simulink library "LibEEPROM_eeprom_example_ORIGINAL"  (Simulink 10.0)
settings: Solver=VariableStepAuto  StartTime=0.0  StopTime=10.0  RelTol=1e-3
undefined symbols (not defined in the file): CRC32_calc_and_EEPROM_Write_ALL, crc32_calc_intern, CRC32_EEPROM_Read, EEPROM_Mirror, EEPROM_Read, IO_Blk_Lib_TTC500, IO_EEPROM_GetStatus, IO_EEPROM_Init, IO_EEPROM_Write, Read_Mirror, Write_Mirror, Write_Mirror_prepare_EEPROM
libraries: simulink x56
(part 7 of 8)

== system LibEEPROM_eeprom_example_ORIGINAL/EEPROM_WriteRetain/EEPROM_retain_var_1 ==
  note: NO IO_EEPROM_Write
      | perfomted here. This is
      | done in CRC32_calc_and_EEPROM_Write_ALL
  trigger : Inport
  data : Inport  Port=2  OutDataTypeStr=EEPROM_type
  Compare To Zero : simulink/Logic and Bit Operations/Compare To Zero  relop===  OutDataTypeStr=boolean  ZeroCross=off
  Compare To Zero1 : simulink/Logic and Bit Operations/Compare To Zero  relop=~=  OutDataTypeStr=boolean  ZeroCross=off
  Write_Mirror : Subsystem  LoadFcn=|  mask(Write_Mirror_Code){SampleTime=-1, ttlib=IO_Blk_Lib_TTC500, ttDescription=Write_Mirror, tt_iolib_version=0.19, offset=offset, length=length}
      | try
      | %
      | %Upgrade Information - standard BEGIN
      | new_color = 'blue';
      | new_ver = '0.19';
      | act_ver = get_param(gcb,'tt_iolib_version');
      | if not(strcmp(act_ver,new_ver))
      |     disp(['Upgrade block: ',gcb,char(10),'       Version: ',act_ver,' -> ',new_ver]);
      |     %switch - case for specific upgrade information e.g. additional parameter required 
      |     %Change appearance and version information
      |     set_param(gcb,'ForegroundColor',new_color);
      |     set_param(gcb,'tt_iolib_version',new_ver);
      | end
      | %Upgrade Information - standard END
      | catch
      | %Standard catch section BEGIN 
      | disp(' ');
      | disp('------------------------------------------------------------');
      | disp('An error occurred in a callback of the TTC580-BlockLib.');
      | disp('Please copy the following lines and report this to support@tttech.com ');
      | disp('<< begin of error message dump >>');
      | disp(['Version of TTC580-BlockLib: ', get_param(gcb,'tt_iolib_version')]);
      | disp(get_param(gcb,'ttDescription'));
      | disp(gcb);
      | x=lasterror;disp(x.message);
      | disp(get_param(gcb,'MaskValues'));
      | disp(version);
      | disp(computer);
      | disp('<< end of error message dump >>');
      | disp('------------------------------------------------------------');
      | disp(' ');
      | %Standard catch section END
      | end
      mask help:
      | Write data to the mirror of the EEPROM. ErrorCode is set to IO_E_BUSY for one cycle of writing into EEPROM_mirror[].
      | In case the given data section exceeds given EEPROM boundaries, IO_E_EEPROM_RANGE ErrorCode is returned.
      mask init:
      | %
      settings: CopyFcn=%deleted
      mask Help: web(which('~.h'))
      mask Callback offset: %
      mask Callback length: %
  b_ready : Outport  VectorParamsAs1DForOutWhenUnconnected=off
  wires:
  Compare To Zero1/1 -> Write_Mirror/1(b_trigger)
  Write_Mirror/1(ErrorCode_EEPROM_mirror) -> Compare To Zero/1
  data/1 -> Write_Mirror/2(data)
  trigger/1 -> Compare To Zero1/1
  Compare To Zero/1 -> b_ready/1

== system LibEEPROM_eeprom_example_ORIGINAL/EEPROM_WriteRetain/EEPROM_retain_var_2 ==
  note: NO IO_EEPROM_Write
      | perfomted here. This is
      | done in CRC32_calc_and_EEPROM_Write_ALL
  trigger : Inport
  data : Inport  Port=2  OutDataTypeStr=EEPROM_type
  Compare To Zero : simulink/Logic and Bit Operations/Compare To Zero  relop===  OutDataTypeStr=boolean  ZeroCross=off
  Compare To Zero1 : simulink/Logic and Bit Operations/Compare To Zero  relop=~=  OutDataTypeStr=boolean  ZeroCross=off
  Write_Mirror : Subsystem  LoadFcn=|  mask(Write_Mirror_Code){SampleTime=-1, ttlib=IO_Blk_Lib_TTC500, ttDescription=Write_Mirror, tt_iolib_version=0.19, offset=offset, length=length}
      | try
      | %
      | %Upgrade Information - standard BEGIN
      | new_color = 'blue';
      | new_ver = '0.19';
      | act_ver = get_param(gcb,'tt_iolib_version');
      | if not(strcmp(act_ver,new_ver))
      |     disp(['Upgrade block: ',gcb,char(10),'       Version: ',act_ver,' -> ',new_ver]);
      |     %switch - case for specific upgrade information e.g. additional parameter required 
      |     %Change appearance and version information
      |     set_param(gcb,'ForegroundColor',new_color);
      |     set_param(gcb,'tt_iolib_version',new_ver);
      | end
      | %Upgrade Information - standard END
      | catch
      | %Standard catch section BEGIN 
      | disp(' ');
      | disp('------------------------------------------------------------');
      | disp('An error occurred in a callback of the TTC580-BlockLib.');
      | disp('Please copy the following lines and report this to support@tttech.com ');
      | disp('<< begin of error message dump >>');
      | disp(['Version of TTC580-BlockLib: ', get_param(gcb,'tt_iolib_version')]);
      | disp(get_param(gcb,'ttDescription'));
      | disp(gcb);
      | x=lasterror;disp(x.message);
      | disp(get_param(gcb,'MaskValues'));
      | disp(version);
      | disp(computer);
      | disp('<< end of error message dump >>');
      | disp('------------------------------------------------------------');
      | disp(' ');
      | %Standard catch section END
      | end
      mask help:
      | Write data to the mirror of the EEPROM. ErrorCode is set to IO_E_BUSY for one cycle of writing into EEPROM_mirror[].
      | In case the given data section exceeds given EEPROM boundaries, IO_E_EEPROM_RANGE ErrorCode is returned.
      mask init:
      | %
      settings: CopyFcn=%deleted
      mask Help: web(which('~.h'))
      mask Callback offset: %
      mask Callback length: %
  b_ready : Outport  VectorParamsAs1DForOutWhenUnconnected=off
  wires:
  Compare To Zero1/1 -> Write_Mirror/1(b_trigger)
  Write_Mirror/1(ErrorCode_EEPROM_mirror) -> Compare To Zero/1
  data/1 -> Write_Mirror/2(data)
  trigger/1 -> Compare To Zero1/1
  Compare To Zero/1 -> b_ready/1

== system LibEEPROM_eeprom_example_ORIGINAL/EEPROM_WriteRetain/EEPROM_retain_var_3 ==
  note: NO IO_EEPROM_Write
      | perfomted here. This is
      | done in CRC32_calc_and_EEPROM_Write_ALL
  trigger : Inport
  data : Inport  Port=2  OutDataTypeStr=EEPROM_type
  Compare To Zero : simulink/Logic and Bit Operations/Compare To Zero  relop===  OutDataTypeStr=boolean  ZeroCross=off
  Compare To Zero1 : simulink/Logic and Bit Operations/Compare To Zero  relop=~=  OutDataTypeStr=boolean  ZeroCross=off
  Write_Mirror : Subsystem  LoadFcn=|  mask(Write_Mirror_Code){SampleTime=-1, ttlib=IO_Blk_Lib_TTC500, ttDescription=Write_Mirror, tt_iolib_version=0.19, offset=offset, length=length}
      | try
      | %
      | %Upgrade Information - standard BEGIN
      | new_color = 'blue';
      | new_ver = '0.19';
      | act_ver = get_param(gcb,'tt_iolib_version');
      | if not(strcmp(act_ver,new_ver))
      |     disp(['Upgrade block: ',gcb,char(10),'       Version: ',act_ver,' -> ',new_ver]);
      |     %switch - case for specific upgrade information e.g. additional parameter required 
      |     %Change appearance and version information
      |     set_param(gcb,'ForegroundColor',new_color);
      |     set_param(gcb,'tt_iolib_version',new_ver);
      | end
      | %Upgrade Information - standard END
      | catch
      | %Standard catch section BEGIN 
      | disp(' ');
      | disp('------------------------------------------------------------');
      | disp('An error occurred in a callback of the TTC580-BlockLib.');
      | disp('Please copy the following lines and report this to support@tttech.com ');
      | disp('<< begin of error message dump >>');
      | disp(['Version of TTC580-BlockLib: ', get_param(gcb,'tt_iolib_version')]);
      | disp(get_param(gcb,'ttDescription'));
      | disp(gcb);
      | x=lasterror;disp(x.message);
      | disp(get_param(gcb,'MaskValues'));
      | disp(version);
      | disp(computer);
      | disp('<< end of error message dump >>');
      | disp('------------------------------------------------------------');
      | disp(' ');
      | %Standard catch section END
      | end
      mask help:
      | Write data to the mirror of the EEPROM. ErrorCode is set to IO_E_BUSY for one cycle of writing into EEPROM_mirror[].
      | In case the given data section exceeds given EEPROM boundaries, IO_E_EEPROM_RANGE ErrorCode is returned.
      mask init:
      | %
      settings: CopyFcn=%deleted
      mask Help: web(which('~.h'))
      mask Callback offset: %
      mask Callback length: %
  b_ready : Outport  VectorParamsAs1DForOutWhenUnconnected=off
  wires:
  Compare To Zero1/1 -> Write_Mirror/1(b_trigger)
  Write_Mirror/1(ErrorCode_EEPROM_mirror) -> Compare To Zero/1
  data/1 -> Write_Mirror/2(data)
  trigger/1 -> Compare To Zero1/1
  Compare To Zero/1 -> b_ready/1

== system LibEEPROM_eeprom_example_ORIGINAL/EEPROM_WriteRetain/EEPROM_retain_var_4 ==
  note: NO IO_EEPROM_Write
      | perfomted here. This is
      | done in CRC32_calc_and_EEPROM_Write_ALL
  trigger : Inport
  data : Inport  Port=2  OutDataTypeStr=EEPROM_type
  Compare To Zero : simulink/Logic and Bit Operations/Compare To Zero  relop===  OutDataTypeStr=boolean  ZeroCross=off
  Compare To Zero1 : simulink/Logic and Bit Operations/Compare To Zero  relop=~=  OutDataTypeStr=boolean  ZeroCross=off
  Write_Mirror : Subsystem  LoadFcn=|  mask(Write_Mirror_Code){SampleTime=-1, ttlib=IO_Blk_Lib_TTC500, ttDescription=Write_Mirror, tt_iolib_version=0.19, offset=offset, length=length}
      | try
      | %
      | %Upgrade Information - standard BEGIN
      | new_color = 'blue';
      | new_ver = '0.19';
      | act_ver = get_param(gcb,'tt_iolib_version');
      | if not(strcmp(act_ver,new_ver))
      |     disp(['Upgrade block: ',gcb,char(10),'       Version: ',act_ver,' -> ',new_ver]);
      |     %switch - case for specific upgrade information e.g. additional parameter required 
      |     %Change appearance and version information
      |     set_param(gcb,'ForegroundColor',new_color);
      |     set_param(gcb,'tt_iolib_version',new_ver);
      | end
      | %Upgrade Information - standard END
      | catch
      | %Standard catch section BEGIN 
      | disp(' ');
      | disp('------------------------------------------------------------');
      | disp('An error occurred in a callback of the TTC580-BlockLib.');
      | disp('Please copy the following lines and report this to support@tttech.com ');
      | disp('<< begin of error message dump >>');
      | disp(['Version of TTC580-BlockLib: ', get_param(gcb,'tt_iolib_version')]);
      | disp(get_param(gcb,'ttDescription'));
      | disp(gcb);
      | x=lasterror;disp(x.message);
      | disp(get_param(gcb,'MaskValues'));
      | disp(version);
      | disp(computer);
      | disp('<< end of error message dump >>');
      | disp('------------------------------------------------------------');
      | disp(' ');
      | %Standard catch section END
      | end
      mask help:
      | Write data to the mirror of the EEPROM. ErrorCode is set to IO_E_BUSY for one cycle of writing into EEPROM_mirror[].
      | In case the given data section exceeds given EEPROM boundaries, IO_E_EEPROM_RANGE ErrorCode is returned.
      mask init:
      | %
      settings: CopyFcn=%deleted
      mask Help: web(which('~.h'))
      mask Callback offset: %
      mask Callback length: %
  b_ready : Outport  VectorParamsAs1DForOutWhenUnconnected=off
  wires:
  Compare To Zero1/1 -> Write_Mirror/1(b_trigger)
  Write_Mirror/1(ErrorCode_EEPROM_mirror) -> Compare To Zero/1
  data/1 -> Write_Mirror/2(data)
  trigger/1 -> Compare To Zero1/1
  Compare To Zero/1 -> b_ready/1

== system LibEEPROM_eeprom_example_ORIGINAL/EEPROM_WriteRetain/EEPROM_retain_var_5 ==
  note: NO IO_EEPROM_Write
      | perfomted here. This is
      | done in CRC32_calc_and_EEPROM_Write_ALL
  trigger : Inport
  data : Inport  Port=2  OutDataTypeStr=EEPROM_type
  Compare To Zero : simulink/Logic and Bit Operations/Compare To Zero  relop===  OutDataTypeStr=boolean  ZeroCross=off
  Compare To Zero1 : simulink/Logic and Bit Operations/Compare To Zero  relop=~=  OutDataTypeStr=boolean  ZeroCross=off
  Write_Mirror : Subsystem  LoadFcn=|  mask(Write_Mirror_Code){SampleTime=-1, ttlib=IO_Blk_Lib_TTC500, ttDescription=Write_Mirror, tt_iolib_version=0.19, offset=offset, length=length}
      | try
      | %
      | %Upgrade Information - standard BEGIN
      | new_color = 'blue';
      | new_ver = '0.19';
      | act_ver = get_param(gcb,'tt_iolib_version');
      | if not(strcmp(act_ver,new_ver))
      |     disp(['Upgrade block: ',gcb,char(10),'       Version: ',act_ver,' -> ',new_ver]);
      |     %switch - case for specific upgrade information e.g. additional parameter required 
      |     %Change appearance and version information
      |     set_param(gcb,'ForegroundColor',new_color);
      |     set_param(gcb,'tt_iolib_version',new_ver);
      | end
      | %Upgrade Information - standard END
      | catch
      | %Standard catch section BEGIN 
      | disp(' ');
      | disp('------------------------------------------------------------');
      | disp('An error occurred in a callback of the TTC580-BlockLib.');
      | disp('Please copy the following lines and report this to support@tttech.com ');
      | disp('<< begin of error message dump >>');
      | disp(['Version of TTC580-BlockLib: ', get_param(gcb,'tt_iolib_version')]);
      | disp(get_param(gcb,'ttDescription'));
      | disp(gcb);
      | x=lasterror;disp(x.message);
      | disp(get_param(gcb,'MaskValues'));
      | disp(version);
      | disp(computer);
      | disp('<< end of error message dump >>');
      | disp('------------------------------------------------------------');
      | disp(' ');
      | %Standard catch section END
      | end
      mask help:
      | Write data to the mirror of the EEPROM. ErrorCode is set to IO_E_BUSY for one cycle of writing into EEPROM_mirror[].
      | In case the given data section exceeds given EEPROM boundaries, IO_E_EEPROM_RANGE ErrorCode is returned.
      mask init:
      | %
      settings: CopyFcn=%deleted
      mask Help: web(which('~.h'))
      mask Callback offset: %
      mask Callback length: %
  b_ready : Outport  VectorParamsAs1DForOutWhenUnconnected=off
  wires:
  Compare To Zero1/1 -> Write_Mirror/1(b_trigger)
  Write_Mirror/1(ErrorCode_EEPROM_mirror) -> Compare To Zero/1
  data/1 -> Write_Mirror/2(data)
  trigger/1 -> Compare To Zero1/1
  Compare To Zero/1 -> b_ready/1

== system LibEEPROM_eeprom_example_ORIGINAL/EEPROM_ReadParam1/EEPROM_CRC_OK/EEPROM_Mirror ==
  EC_EEPROM_Init : Inport
  EEPROM_Mirror_s : S-Function  FunctionName=EEPROM_Mirror_s  Parameters=SampleTime,offset,length  SFunctionDeploymentMode=off  EnableBusSupport=off
  Terminator : Terminator
  wires:
  EC_EEPROM_Init/1 -> EEPROM_Mirror_s/1
  EEPROM_Mirror_s/1 -> Terminator/1

== system LibEEPROM_eeprom_example_ORIGINAL/EEPROM_ReadParam1/EEPROM_CRC_OK/IO_EEPROM_GetStatus ==
  IO_EEPROM_GetStatus_s : S-Function  FunctionName=IO_EEPROM_GetStatus_s  Parameters=SampleTime  SFunctionDeploymentMode=off  EnableBusSupport=off
  ErrorCode : Outport  VectorParamsAs1DForOutWhenUnconnected=off
  wires:
  IO_EEPROM_GetStatus_s/1 -> ErrorCode/1

== system LibEEPROM_eeprom_example_ORIGINAL/EEPROM_ReadParam1/EEPROM_CRC_OK/IO_EEPROM_Init ==
  IO_EEPROM_Init_s : S-Function  FunctionName=IO_EEPROM_Init_s  Parameters=SampleTime  SFunctionDeploymentMode=off  EnableBusSupport=off
  ErrorCode : Outport  VectorParamsAs1DForOutWhenUnconnected=off
  wires:
  IO_EEPROM_Init_s/1 -> ErrorCode/1

== system LibEEPROM_eeprom_example_ORIGINAL/EEPROM_ReadParam1/EEPROM_CRC_OK/Read_Mirror ==
  Read_Mirror_s : S-Function  FunctionName=Read_Mirror_s  Parameters=SampleTime,offset,length  SFunctionDeploymentMode=off  EnableBusSupport=off
  ErrorCode_EEPROM_mirror : Outport  VectorParamsAs1DForOutWhenUnconnected=off
  data : Outport  Port=2  VectorParamsAs1DForOutWhenUnconnected=off
  wires:
  Read_Mirror_s/1 -> ErrorCode_EEPROM_mirror/1
  Read_Mirror_s/2 -> data/1

== system LibEEPROM_eeprom_example_ORIGINAL/EEPROM_ReadParam1/EEPROM_CRC_OK/check & freeze ==
  check1 : Inport
  b_enable : Inport  Port=2
  check2 : Inport  Port=3
  Trigger : TriggerPort  VariantControl=(inherit)
  Logical Operator1 : Logic  AllPortsSameDT=off  OutDataTypeStr=boolean
  Relational Operator : RelationalOperator  Operator===  OutDataTypeStr=boolean  RndMeth=Nearest
  Out : Outport  InitialOutput=0  VectorParamsAs1DForOutWhenUnconnected=off
  wires:
  check2/1 -> Relational Operator/2
  b_enable/1 -> Logical Operator1/2
  Logical Operator1/1 -> Out/1
  check1/1 -> Relational Operator/1
  Relational Operator/1 -> Logical Operator1/1

== system LibEEPROM_eeprom_example_ORIGINAL/EEPROM_ReadParam1/EEPROM_CRC_OK/crc32_calc_intern ==
  Trigger : TriggerPort  VariantControl=(inherit)
  crc32_calc_intern_s : S-Function  FunctionName=crc32_calc_intern_s  Parameters=SampleTime,EEPROM_mirror,iBasicAddr_intern,iEndAddr_intern  SFunctionDeploymentMode=off  EnableBusSupport=off
  ErrorCode : Outport  VectorParamsAs1DForOutWhenUnconnected=off
  crc32 : Outport  Port=2  VectorParamsAs1DForOutWhenUnconnected=off
  wires:
  crc32_calc_intern_s/1 -> ErrorCode/1
  crc32_calc_intern_s/2 -> crc32/1

== system LibEEPROM_eeprom_example_ORIGINAL/EEPROM_ReadParam1/EEPROM_CRC_OK/once_true: Mirror filled ==
  S : Inport
  Logic : CombinatorialLogic  TruthTable=[0 ;1 ;0 ;0 ;1 ;1 ;0 ;0 ]
  Memory : Memory  InitialCondition=initial_condition  InheritSampleTime=on
  Mux : Mux  Inputs=3
  R : Constant  Value=0  OutDataTypeStr=boolean
  Q : Outport  InitialOutput=0  VectorParamsAs1DForOutWhenUnconnected=off
  wires:
  Memory/1 -> Mux/3
  Mux/1 -> Logic/1
  Logic/1 -> Q/1, Memory/1
  S/1 -> Mux/1
  R/1 -> Mux/2

== system LibEEPROM_eeprom_example_ORIGINAL/EEPROM_ReadParam1/EEPROM_param_1/EEPROM_Mirror ==
  EC_EEPROM_Init : Inport
  EEPROM_Mirror_s : S-Function  FunctionName=EEPROM_Mirror_s  Parameters=SampleTime,offset,length  SFunctionDeploymentMode=off  EnableBusSupport=off
  Terminator : Terminator
  wires:
  EC_EEPROM_Init/1 -> EEPROM_Mirror_s/1
  EEPROM_Mirror_s/1 -> Terminator/1

== system LibEEPROM_eeprom_example_ORIGINAL/EEPROM_ReadParam1/EEPROM_param_1/IO_EEPROM_GetStatus ==
  IO_EEPROM_GetStatus_s : S-Function  FunctionName=IO_EEPROM_GetStatus_s  Parameters=SampleTime  SFunctionDeploymentMode=off  EnableBusSupport=off
  ErrorCode : Outport  VectorParamsAs1DForOutWhenUnconnected=off
  wires:
  IO_EEPROM_GetStatus_s/1 -> ErrorCode/1

== system LibEEPROM_eeprom_example_ORIGINAL/EEPROM_ReadParam1/EEPROM_param_1/IO_EEPROM_Init ==
  IO_EEPROM_Init_s : S-Function  FunctionName=IO_EEPROM_Init_s  Parameters=SampleTime  SFunctionDeploymentMode=off  EnableBusSupport=off
  ErrorCode : Outport  VectorParamsAs1DForOutWhenUnconnected=off
  wires:
  IO_EEPROM_Init_s/1 -> ErrorCode/1

== system LibEEPROM_eeprom_example_ORIGINAL/EEPROM_ReadParam1/EEPROM_param_1/Read_Mirror ==
  Read_Mirror_s : S-Function  FunctionName=Read_Mirror_s  Parameters=SampleTime,offset,length  SFunctionDeploymentMode=off  EnableBusSupport=off
  ErrorCode_EEPROM_mirror : Outport  VectorParamsAs1DForOutWhenUnconnected=off
  data : Outport  Port=2  VectorParamsAs1DForOutWhenUnconnected=off
  wires:
  Read_Mirror_s/2 -> data/1
  Read_Mirror_s/1 -> ErrorCode_EEPROM_mirror/1

== system LibEEPROM_eeprom_example_ORIGINAL/EEPROM_ReadParam1/EEPROM_param_1/once_true: Mirror filled ==
  S : Inport
  Logic : CombinatorialLogic  TruthTable=[0 ;1 ;0 ;0 ;1 ;1 ;0 ;0 ]
  Memory : Memory  InitialCondition=initial_condition  InheritSampleTime=on
  Mux : Mux  Inputs=3
  R : Constant  Value=0  OutDataTypeStr=boolean
  Q : Outport  InitialOutput=0  VectorParamsAs1DForOutWhenUnconnected=off
  wires:
  R/1 -> Mux/2
  S/1 -> Mux/1
  Logic/1 -> Memory/1, Q/1
  Mux/1 -> Logic/1
  Memory/1 -> Mux/3

== system LibEEPROM_eeprom_example_ORIGINAL/EEPROM_ReadParam1/EEPROM_param_2/EEPROM_Mirror ==
  EC_EEPROM_Init : Inport
  EEPROM_Mirror_s : S-Function  FunctionName=EEPROM_Mirror_s  Parameters=SampleTime,offset,length  SFunctionDeploymentMode=off  EnableBusSupport=off
  Terminator : Terminator
  wires:
  EC_EEPROM_Init/1 -> EEPROM_Mirror_s/1
  EEPROM_Mirror_s/1 -> Terminator/1

== system LibEEPROM_eeprom_example_ORIGINAL/EEPROM_ReadParam1/EEPROM_param_2/IO_EEPROM_GetStatus ==
  IO_EEPROM_GetStatus_s : S-Function  FunctionName=IO_EEPROM_GetStatus_s  Parameters=SampleTime  SFunctionDeploymentMode=off  EnableBusSupport=off
  ErrorCode : Outport  VectorParamsAs1DForOutWhenUnconnected=off
  wires:
  IO_EEPROM_GetStatus_s/1 -> ErrorCode/1

== system LibEEPROM_eeprom_example_ORIGINAL/EEPROM_ReadParam1/EEPROM_param_2/IO_EEPROM_Init ==
  IO_EEPROM_Init_s : S-Function  FunctionName=IO_EEPROM_Init_s  Parameters=SampleTime  SFunctionDeploymentMode=off  EnableBusSupport=off
  ErrorCode : Outport  VectorParamsAs1DForOutWhenUnconnected=off
  wires:
  IO_EEPROM_Init_s/1 -> ErrorCode/1

== system LibEEPROM_eeprom_example_ORIGINAL/EEPROM_ReadParam1/EEPROM_param_2/Read_Mirror ==
  Read_Mirror_s : S-Function  FunctionName=Read_Mirror_s  Parameters=SampleTime,offset,length  SFunctionDeploymentMode=off  EnableBusSupport=off
  ErrorCode_EEPROM_mirror : Outport  VectorParamsAs1DForOutWhenUnconnected=off
  data : Outport  Port=2  VectorParamsAs1DForOutWhenUnconnected=off
  wires:
  Read_Mirror_s/2 -> data/1
  Read_Mirror_s/1 -> ErrorCode_EEPROM_mirror/1

== system LibEEPROM_eeprom_example_ORIGINAL/EEPROM_ReadParam1/EEPROM_param_2/once_true: Mirror filled ==
  S : Inport
  Logic : CombinatorialLogic  TruthTable=[0 ;1 ;0 ;0 ;1 ;1 ;0 ;0 ]
  Memory : Memory  InitialCondition=initial_condition  InheritSampleTime=on
  Mux : Mux  Inputs=3
  R : Constant  Value=0  OutDataTypeStr=boolean
  Q : Outport  InitialOutput=0  VectorParamsAs1DForOutWhenUnconnected=off
  wires:
  R/1 -> Mux/2
  S/1 -> Mux/1
  Logic/1 -> Memory/1, Q/1
  Mux/1 -> Logic/1
  Memory/1 -> Mux/3

== system LibEEPROM_eeprom_example_ORIGINAL/EEPROM_ReadParam1/EEPROM_param_3/EEPROM_Mirror ==
  EC_EEPROM_Init : Inport
  EEPROM_Mirror_s : S-Function  FunctionName=EEPROM_Mirror_s  Parameters=SampleTime,offset,length  SFunctionDeploymentMode=off  EnableBusSupport=off
  Terminator : Terminator
  wires:
  EC_EEPROM_Init/1 -> EEPROM_Mirror_s/1
  EEPROM_Mirror_s/1 -> Terminator/1

== system LibEEPROM_eeprom_example_ORIGINAL/EEPROM_ReadParam1/EEPROM_param_3/IO_EEPROM_GetStatus ==
  IO_EEPROM_GetStatus_s : S-Function  FunctionName=IO_EEPROM_GetStatus_s  Parameters=SampleTime  SFunctionDeploymentMode=off  EnableBusSupport=off
  ErrorCode : Outport  VectorParamsAs1DForOutWhenUnconnected=off
  wires:
  IO_EEPROM_GetStatus_s/1 -> ErrorCode/1

== system LibEEPROM_eeprom_example_ORIGINAL/EEPROM_ReadParam1/EEPROM_param_3/IO_EEPROM_Init ==
  IO_EEPROM_Init_s : S-Function  FunctionName=IO_EEPROM_Init_s  Parameters=SampleTime  SFunctionDeploymentMode=off  EnableBusSupport=off
  ErrorCode : Outport  VectorParamsAs1DForOutWhenUnconnected=off
  wires:
  IO_EEPROM_Init_s/1 -> ErrorCode/1

== system LibEEPROM_eeprom_example_ORIGINAL/EEPROM_ReadParam1/EEPROM_param_3/Read_Mirror ==
  Read_Mirror_s : S-Function  FunctionName=Read_Mirror_s  Parameters=SampleTime,offset,length  SFunctionDeploymentMode=off  EnableBusSupport=off
  ErrorCode_EEPROM_mirror : Outport  VectorParamsAs1DForOutWhenUnconnected=off
  data : Outport  Port=2  VectorParamsAs1DForOutWhenUnconnected=off
  wires:
  Read_Mirror_s/2 -> data/1
  Read_Mirror_s/1 -> ErrorCode_EEPROM_mirror/1

== system LibEEPROM_eeprom_example_ORIGINAL/EEPROM_ReadParam1/EEPROM_param_3/once_true: Mirror filled ==
  S : Inport
  Logic : CombinatorialLogic  TruthTable=[0 ;1 ;0 ;0 ;1 ;1 ;0 ;0 ]
  Memory : Memory  InitialCondition=initial_condition  InheritSampleTime=on
  Mux : Mux  Inputs=3
  R : Constant  Value=0  OutDataTypeStr=boolean
  Q : Outport  InitialOutput=0  VectorParamsAs1DForOutWhenUnconnected=off
  wires:
  R/1 -> Mux/2
  S/1 -> Mux/1
  Logic/1 -> Memory/1, Q/1
  Mux/1 -> Logic/1
  Memory/1 -> Mux/3

== system LibEEPROM_eeprom_example_ORIGINAL/EEPROM_ReadParam1/EEPROM_param_4/EEPROM_Mirror ==
  EC_EEPROM_Init : Inport
  EEPROM_Mirror_s : S-Function  FunctionName=EEPROM_Mirror_s  Parameters=SampleTime,offset,length  SFunctionDeploymentMode=off  EnableBusSupport=off
  Terminator : Terminator
  wires:
  EC_EEPROM_Init/1 -> EEPROM_Mirror_s/1
  EEPROM_Mirror_s/1 -> Terminator/1

== system LibEEPROM_eeprom_example_ORIGINAL/EEPROM_ReadParam1/EEPROM_param_4/IO_EEPROM_GetStatus ==
  IO_EEPROM_GetStatus_s : S-Function  FunctionName=IO_EEPROM_GetStatus_s  Parameters=SampleTime  SFunctionDeploymentMode=off  EnableBusSupport=off
  ErrorCode : Outport  VectorParamsAs1DForOutWhenUnconnected=off
  wires:
  IO_EEPROM_GetStatus_s/1 -> ErrorCode/1

== system LibEEPROM_eeprom_example_ORIGINAL/EEPROM_ReadParam1/EEPROM_param_4/IO_EEPROM_Init ==
  IO_EEPROM_Init_s : S-Function  FunctionName=IO_EEPROM_Init_s  Parameters=SampleTime  SFunctionDeploymentMode=off  EnableBusSupport=off
  ErrorCode : Outport  VectorParamsAs1DForOutWhenUnconnected=off
  wires:
  IO_EEPROM_Init_s/1 -> ErrorCode/1

== system LibEEPROM_eeprom_example_ORIGINAL/EEPROM_ReadParam1/EEPROM_param_4/Read_Mirror ==
  Read_Mirror_s : S-Function  FunctionName=Read_Mirror_s  Parameters=SampleTime,offset,length  SFunctionDeploymentMode=off  EnableBusSupport=off
  ErrorCode_EEPROM_mirror : Outport  VectorParamsAs1DForOutWhenUnconnected=off
  data : Outport  Port=2  VectorParamsAs1DForOutWhenUnconnected=off
  wires:
  Read_Mirror_s/2 -> data/1
  Read_Mirror_s/1 -> ErrorCode_EEPROM_mirror/1

== system LibEEPROM_eeprom_example_ORIGINAL/EEPROM_ReadParam1/EEPROM_param_4/once_true: Mirror filled ==
  S : Inport
  Logic : CombinatorialLogic  TruthTable=[0 ;1 ;0 ;0 ;1 ;1 ;0 ;0 ]
  Memory : Memory  InitialCondition=initial_condition  InheritSampleTime=on
  Mux : Mux  Inputs=3
  R : Constant  Value=0  OutDataTypeStr=boolean
  Q : Outport  InitialOutput=0  VectorParamsAs1DForOutWhenUnconnected=off
  wires:
  R/1 -> Mux/2
  S/1 -> Mux/1
  Logic/1 -> Memory/1, Q/1
  Mux/1 -> Logic/1
  Memory/1 -> Mux/3

== system LibEEPROM_eeprom_example_ORIGINAL/EEPROM_ReadParam1/EEPROM_param_5/EEPROM_Mirror ==
  EC_EEPROM_Init : Inport
  EEPROM_Mirror_s : S-Function  FunctionName=EEPROM_Mirror_s  Parameters=SampleTime,offset,length  SFunctionDeploymentMode=off  EnableBusSupport=off
  Terminator : Terminator
  wires:
  EC_EEPROM_Init/1 -> EEPROM_Mirror_s/1
  EEPROM_Mirror_s/1 -> Terminator/1

== system LibEEPROM_eeprom_example_ORIGINAL/EEPROM_ReadParam1/EEPROM_param_5/IO_EEPROM_GetStatus ==
  IO_EEPROM_GetStatus_s : S-Function  FunctionName=IO_EEPROM_GetStatus_s  Parameters=SampleTime  SFunctionDeploymentMode=off  EnableBusSupport=off
  ErrorCode : Outport  VectorParamsAs1DForOutWhenUnconnected=off
  wires:
  IO_EEPROM_GetStatus_s/1 -> ErrorCode/1

== system LibEEPROM_eeprom_example_ORIGINAL/EEPROM_ReadParam1/EEPROM_param_5/IO_EEPROM_Init ==
  IO_EEPROM_Init_s : S-Function  FunctionName=IO_EEPROM_Init_s  Parameters=SampleTime  SFunctionDeploymentMode=off  EnableBusSupport=off
  ErrorCode : Outport  VectorParamsAs1DForOutWhenUnconnected=off
  wires:
  IO_EEPROM_Init_s/1 -> ErrorCode/1

== system LibEEPROM_eeprom_example_ORIGINAL/EEPROM_ReadParam1/EEPROM_param_5/Read_Mirror ==
  Read_Mirror_s : S-Function  FunctionName=Read_Mirror_s  Parameters=SampleTime,offset,length  SFunctionDeploymentMode=off  EnableBusSupport=off
  ErrorCode_EEPROM_mirror : Outport  VectorParamsAs1DForOutWhenUnconnected=off
  data : Outport  Port=2  VectorParamsAs1DForOutWhenUnconnected=off
  wires:
  Read_Mirror_s/2 -> data/1
  Read_Mirror_s/1 -> ErrorCode_EEPROM_mirror/1

== system LibEEPROM_eeprom_example_ORIGINAL/EEPROM_ReadParam1/EEPROM_param_5/once_true: Mirror filled ==
  S : Inport
  Logic : CombinatorialLogic  TruthTable=[0 ;1 ;0 ;0 ;1 ;1 ;0 ;0 ]
  Memory : Memory  InitialCondition=initial_condition  InheritSampleTime=on
  Mux : Mux  Inputs=3
  R : Constant  Value=0  OutDataTypeStr=boolean
  Q : Outport  InitialOutput=0  VectorParamsAs1DForOutWhenUnconnected=off
  wires:
  R/1 -> Mux/2
  S/1 -> Mux/1
  Logic/1 -> Memory/1, Q/1
  Mux/1 -> Logic/1
  Memory/1 -> Mux/3

== system LibEEPROM_eeprom_example_ORIGINAL/EEPROM_ReadParam1/EEPROM_param_6/EEPROM_Mirror ==
  EC_EEPROM_Init : Inport
  EEPROM_Mirror_s : S-Function  FunctionName=EEPROM_Mirror_s  Parameters=SampleTime,offset,length  SFunctionDeploymentMode=off  EnableBusSupport=off
  Terminator : Terminator
  wires:
  EC_EEPROM_Init/1 -> EEPROM_Mirror_s/1
  EEPROM_Mirror_s/1 -> Terminator/1

== system LibEEPROM_eeprom_example_ORIGINAL/EEPROM_ReadParam1/EEPROM_param_6/IO_EEPROM_GetStatus ==
  IO_EEPROM_GetStatus_s : S-Function  FunctionName=IO_EEPROM_GetStatus_s  Parameters=SampleTime  SFunctionDeploymentMode=off  EnableBusSupport=off
  ErrorCode : Outport  VectorParamsAs1DForOutWhenUnconnected=off
  wires:
  IO_EEPROM_GetStatus_s/1 -> ErrorCode/1

== system LibEEPROM_eeprom_example_ORIGINAL/EEPROM_ReadParam1/EEPROM_param_6/IO_EEPROM_Init ==
  IO_EEPROM_Init_s : S-Function  FunctionName=IO_EEPROM_Init_s  Parameters=SampleTime  SFunctionDeploymentMode=off  EnableBusSupport=off
  ErrorCode : Outport  VectorParamsAs1DForOutWhenUnconnected=off
  wires:
  IO_EEPROM_Init_s/1 -> ErrorCode/1

== system LibEEPROM_eeprom_example_ORIGINAL/EEPROM_ReadParam1/EEPROM_param_6/Read_Mirror ==
  Read_Mirror_s : S-Function  FunctionName=Read_Mirror_s  Parameters=SampleTime,offset,length  SFunctionDeploymentMode=off  EnableBusSupport=off
  ErrorCode_EEPROM_mirror : Outport  VectorParamsAs1DForOutWhenUnconnected=off
  data : Outport  Port=2  VectorParamsAs1DForOutWhenUnconnected=off
  wires:
  Read_Mirror_s/2 -> data/1
  Read_Mirror_s/1 -> ErrorCode_EEPROM_mirror/1

== system LibEEPROM_eeprom_example_ORIGINAL/EEPROM_ReadParam1/EEPROM_param_6/once_true: Mirror filled ==
  S : Inport
  Logic : CombinatorialLogic  TruthTable=[0 ;1 ;0 ;0 ;1 ;1 ;0 ;0 ]
  Memory : Memory  InitialCondition=initial_condition  InheritSampleTime=on
  Mux : Mux  Inputs=3
  R : Constant  Value=0  OutDataTypeStr=boolean
  Q : Outport  InitialOutput=0  VectorParamsAs1DForOutWhenUnconnected=off
  wires:
  R/1 -> Mux/2
  S/1 -> Mux/1
  Logic/1 -> Memory/1, Q/1
  Mux/1 -> Logic/1
  Memory/1 -> Mux/3

== system LibEEPROM_eeprom_example_ORIGINAL/EEPROM_ReadRetain/EEPROM_CRC_OK/EEPROM_Mirror ==
  EC_EEPROM_Init : Inport
  EEPROM_Mirror_s : S-Function  FunctionName=EEPROM_Mirror_s  Parameters=SampleTime,offset,length  SFunctionDeploymentMode=off  EnableBusSupport=off
  Terminator : Terminator
  wires:
  EC_EEPROM_Init/1 -> EEPROM_Mirror_s/1
  EEPROM_Mirror_s/1 -> Terminator/1

== system LibEEPROM_eeprom_example_ORIGINAL/EEPROM_ReadRetain/EEPROM_CRC_OK/IO_EEPROM_GetStatus ==
  IO_EEPROM_GetStatus_s : S-Function  FunctionName=IO_EEPROM_GetStatus_s  Parameters=SampleTime  SFunctionDeploymentMode=off  EnableBusSupport=off
  ErrorCode : Outport  VectorParamsAs1DForOutWhenUnconnected=off
  wires:
  IO_EEPROM_GetStatus_s/1 -> ErrorCode/1

== system LibEEPROM_eeprom_example_ORIGINAL/EEPROM_ReadRetain/EEPROM_CRC_OK/IO_EEPROM_Init ==
  IO_EEPROM_Init_s : S-Function  FunctionName=IO_EEPROM_Init_s  Parameters=SampleTime  SFunctionDeploymentMode=off  EnableBusSupport=off
  ErrorCode : Outport  VectorParamsAs1DForOutWhenUnconnected=off
  wires:
  IO_EEPROM_Init_s/1 -> ErrorCode/1

== system LibEEPROM_eeprom_example_ORIGINAL/EEPROM_ReadRetain/EEPROM_CRC_OK/Read_Mirror ==
  Read_Mirror_s : S-Function  FunctionName=Read_Mirror_s  Parameters=SampleTime,offset,length  SFunctionDeploymentMode=off  EnableBusSupport=off
  ErrorCode_EEPROM_mirror : Outport  VectorParamsAs1DForOutWhenUnconnected=off
  data : Outport  Port=2  VectorParamsAs1DForOutWhenUnconnected=off
  wires:
  Read_Mirror_s/1 -> ErrorCode_EEPROM_mirror/1
  Read_Mirror_s/2 -> data/1

== system LibEEPROM_eeprom_example_ORIGINAL/EEPROM_ReadRetain/EEPROM_CRC_OK/check & freeze ==
  check1 : Inport
  b_enable : Inport  Port=2
  check2 : Inport  Port=3
  Trigger : TriggerPort  VariantControl=(inherit)
  Logical Operator1 : Logic  AllPortsSameDT=off  OutDataTypeStr=boolean
  Relational Operator : RelationalOperator  Operator===  OutDataTypeStr=boolean  RndMeth=Nearest
  Out : Outport  InitialOutput=0  VectorParamsAs1DForOutWhenUnconnected=off
  wires:
  check2/1 -> Relational Operator/2
  b_enable/1 -> Logical Operator1/2
  Logical Operator1/1 -> Out/1
  check1/1 -> Relational Operator/1
  Relational Operator/1 -> Logical Operator1/1

== system LibEEPROM_eeprom_example_ORIGINAL/EEPROM_ReadRetain/EEPROM_CRC_OK/crc32_calc_intern ==
  Trigger : TriggerPort  VariantControl=(inherit)
  crc32_calc_intern_s : S-Function  FunctionName=crc32_calc_intern_s  Parameters=SampleTime,EEPROM_mirror,iBasicAddr_intern,iEndAddr_intern  SFunctionDeploymentMode=off  EnableBusSupport=off
  ErrorCode : Outport  VectorParamsAs1DForOutWhenUnconnected=off
  crc32 : Outport  Port=2  VectorParamsAs1DForOutWhenUnconnected=off
  wires:
  crc32_calc_intern_s/1 -> ErrorCode/1
  crc32_calc_intern_s/2 -> crc32/1

== system LibEEPROM_eeprom_example_ORIGINAL/EEPROM_ReadRetain/EEPROM_CRC_OK/once_true: Mirror filled ==
  S : Inport
  Logic : CombinatorialLogic  TruthTable=[0 ;1 ;0 ;0 ;1 ;1 ;0 ;0 ]
  Memory : Memory  InitialCondition=initial_condition  InheritSampleTime=on
  Mux : Mux  Inputs=3
  R : Constant  Value=0  OutDataTypeStr=boolean
  Q : Outport  InitialOutput=0  VectorParamsAs1DForOutWhenUnconnected=off
  wires:
  Memory/1 -> Mux/3
  Mux/1 -> Logic/1
  Logic/1 -> Q/1, Memory/1
  S/1 -> Mux/1
  R/1 -> Mux/2

== system LibEEPROM_eeprom_example_ORIGINAL/EEPROM_ReadRetain/EEPROM_retain_var_1/EEPROM_Mirror ==
  EC_EEPROM_Init : Inport
  EEPROM_Mirror_s : S-Function  FunctionName=EEPROM_Mirror_s  Parameters=SampleTime,offset,length  SFunctionDeploymentMode=off  EnableBusSupport=off
  Terminator : Terminator
  wires:
  EC_EEPROM_Init/1 -> EEPROM_Mirror_s/1
  EEPROM_Mirror_s/1 -> Terminator/1

== system LibEEPROM_eeprom_example_ORIGINAL/EEPROM_ReadRetain/EEPROM_retain_var_1/IO_EEPROM_GetStatus ==
  IO_EEPROM_GetStatus_s : S-Function  FunctionName=IO_EEPROM_GetStatus_s  Parameters=SampleTime  SFunctionDeploymentMode=off  EnableBusSupport=off
  ErrorCode : Outport  VectorParamsAs1DForOutWhenUnconnected=off
  wires:
  IO_EEPROM_GetStatus_s/1 -> ErrorCode/1

== system LibEEPROM_eeprom_example_ORIGINAL/EEPROM_ReadRetain/EEPROM_retain_var_1/IO_EEPROM_Init ==
  IO_EEPROM_Init_s : S-Function  FunctionName=IO_EEPROM_Init_s  Parameters=SampleTime  SFunctionDeploymentMode=off  EnableBusSupport=off
  ErrorCode : Outport  VectorParamsAs1DForOutWhenUnconnected=off
  wires:
  IO_EEPROM_Init_s/1 -> ErrorCode/1

== system LibEEPROM_eeprom_example_ORIGINAL/EEPROM_ReadRetain/EEPROM_retain_var_1/Read_Mirror ==
  Read_Mirror_s : S-Function  FunctionName=Read_Mirror_s  Parameters=SampleTime,offset,length  SFunctionDeploymentMode=off  EnableBusSupport=off
  ErrorCode_EEPROM_mirror : Outport  VectorParamsAs1DForOutWhenUnconnected=off
  data : Outport  Port=2  VectorParamsAs1DForOutWhenUnconnected=off
  wires:
  Read_Mirror_s/2 -> data/1
  Read_Mirror_s/1 -> ErrorCode_EEPROM_mirror/1

== system LibEEPROM_eeprom_example_ORIGINAL/EEPROM_ReadRetain/EEPROM_retain_var_1/once_true: Mirror filled ==
  S : Inport
  Logic : CombinatorialLogic  TruthTable=[0 ;1 ;0 ;0 ;1 ;1 ;0 ;0 ]
  Memory : Memory  InitialCondition=initial_condition  InheritSampleTime=on
  Mux : Mux  Inputs=3
  R : Constant  Value=0  OutDataTypeStr=boolean
  Q : Outport  InitialOutput=0  VectorParamsAs1DForOutWhenUnconnected=off
  wires:
  R/1 -> Mux/2
  S/1 -> Mux/1
  Logic/1 -> Memory/1, Q/1
  Mux/1 -> Logic/1
  Memory/1 -> Mux/3

== system LibEEPROM_eeprom_example_ORIGINAL/EEPROM_ReadRetain/EEPROM_retain_var_2/EEPROM_Mirror ==
  EC_EEPROM_Init : Inport
  EEPROM_Mirror_s : S-Function  FunctionName=EEPROM_Mirror_s  Parameters=SampleTime,offset,length  SFunctionDeploymentMode=off  EnableBusSupport=off
  Terminator : Terminator
  wires:
  EC_EEPROM_Init/1 -> EEPROM_Mirror_s/1
  EEPROM_Mirror_s/1 -> Terminator/1

== system LibEEPROM_eeprom_example_ORIGINAL/EEPROM_ReadRetain/EEPROM_retain_var_2/IO_EEPROM_GetStatus ==
  IO_EEPROM_GetStatus_s : S-Function  FunctionName=IO_EEPROM_GetStatus_s  Parameters=SampleTime  SFunctionDeploymentMode=off  EnableBusSupport=off
  ErrorCode : Outport  VectorParamsAs1DForOutWhenUnconnected=off
  wires:
  IO_EEPROM_GetStatus_s/1 -> ErrorCode/1

== system LibEEPROM_eeprom_example_ORIGINAL/EEPROM_ReadRetain/EEPROM_retain_var_2/IO_EEPROM_Init ==
  IO_EEPROM_Init_s : S-Function  FunctionName=IO_EEPROM_Init_s  Parameters=SampleTime  SFunctionDeploymentMode=off  EnableBusSupport=off
  ErrorCode : Outport  VectorParamsAs1DForOutWhenUnconnected=off
  wires:
  IO_EEPROM_Init_s/1 -> ErrorCode/1

== system LibEEPROM_eeprom_example_ORIGINAL/EEPROM_ReadRetain/EEPROM_retain_var_2/Read_Mirror ==
  Read_Mirror_s : S-Function  FunctionName=Read_Mirror_s  Parameters=SampleTime,offset,length  SFunctionDeploymentMode=off  EnableBusSupport=off
  ErrorCode_EEPROM_mirror : Outport  VectorParamsAs1DForOutWhenUnconnected=off
  data : Outport  Port=2  VectorParamsAs1DForOutWhenUnconnected=off
  wires:
  Read_Mirror_s/2 -> data/1
  Read_Mirror_s/1 -> ErrorCode_EEPROM_mirror/1

== system LibEEPROM_eeprom_example_ORIGINAL/EEPROM_ReadRetain/EEPROM_retain_var_2/once_true: Mirror filled ==
  S : Inport
  Logic : CombinatorialLogic  TruthTable=[0 ;1 ;0 ;0 ;1 ;1 ;0 ;0 ]
  Memory : Memory  InitialCondition=initial_condition  InheritSampleTime=on
  Mux : Mux  Inputs=3
  R : Constant  Value=0  OutDataTypeStr=boolean
  Q : Outport  InitialOutput=0  VectorParamsAs1DForOutWhenUnconnected=off
  wires:
  R/1 -> Mux/2
  S/1 -> Mux/1
  Logic/1 -> Memory/1, Q/1
  Mux/1 -> Logic/1
  Memory/1 -> Mux/3

== system LibEEPROM_eeprom_example_ORIGINAL/EEPROM_ReadRetain/EEPROM_retain_var_3/EEPROM_Mirror ==
  EC_EEPROM_Init : Inport
  EEPROM_Mirror_s : S-Function  FunctionName=EEPROM_Mirror_s  Parameters=SampleTime,offset,length  SFunctionDeploymentMode=off  EnableBusSupport=off
  Terminator : Terminator
  wires:
  EC_EEPROM_Init/1 -> EEPROM_Mirror_s/1
  EEPROM_Mirror_s/1 -> Terminator/1

== system LibEEPROM_eeprom_example_ORIGINAL/EEPROM_ReadRetain/EEPROM_retain_var_3/IO_EEPROM_GetStatus ==
  IO_EEPROM_GetStatus_s : S-Function  FunctionName=IO_EEPROM_GetStatus_s  Parameters=SampleTime  SFunctionDeploymentMode=off  EnableBusSupport=off
  ErrorCode : Outport  VectorParamsAs1DForOutWhenUnconnected=off
  wires:
  IO_EEPROM_GetStatus_s/1 -> ErrorCode/1

== system LibEEPROM_eeprom_example_ORIGINAL/EEPROM_ReadRetain/EEPROM_retain_var_3/IO_EEPROM_Init ==
  IO_EEPROM_Init_s : S-Function  FunctionName=IO_EEPROM_Init_s  Parameters=SampleTime  SFunctionDeploymentMode=off  EnableBusSupport=off
  ErrorCode : Outport  VectorParamsAs1DForOutWhenUnconnected=off
  wires:
  IO_EEPROM_Init_s/1 -> ErrorCode/1

== system LibEEPROM_eeprom_example_ORIGINAL/EEPROM_ReadRetain/EEPROM_retain_var_3/Read_Mirror ==
  Read_Mirror_s : S-Function  FunctionName=Read_Mirror_s  Parameters=SampleTime,offset,length  SFunctionDeploymentMode=off  EnableBusSupport=off
  ErrorCode_EEPROM_mirror : Outport  VectorParamsAs1DForOutWhenUnconnected=off
  data : Outport  Port=2  VectorParamsAs1DForOutWhenUnconnected=off
  wires:
  Read_Mirror_s/2 -> data/1
  Read_Mirror_s/1 -> ErrorCode_EEPROM_mirror/1

== system LibEEPROM_eeprom_example_ORIGINAL/EEPROM_ReadRetain/EEPROM_retain_var_3/once_true: Mirror filled ==
  S : Inport
  Logic : CombinatorialLogic  TruthTable=[0 ;1 ;0 ;0 ;1 ;1 ;0 ;0 ]
  Memory : Memory  InitialCondition=initial_condition  InheritSampleTime=on
  Mux : Mux  Inputs=3
  R : Constant  Value=0  OutDataTypeStr=boolean
  Q : Outport  InitialOutput=0  VectorParamsAs1DForOutWhenUnconnected=off
  wires:
  R/1 -> Mux/2
  S/1 -> Mux/1
  Logic/1 -> Memory/1, Q/1
  Mux/1 -> Logic/1
  Memory/1 -> Mux/3

== system LibEEPROM_eeprom_example_ORIGINAL/EEPROM_ReadRetain/EEPROM_retain_var_4/EEPROM_Mirror ==
  EC_EEPROM_Init : Inport
  EEPROM_Mirror_s : S-Function  FunctionName=EEPROM_Mirror_s  Parameters=SampleTime,offset,length  SFunctionDeploymentMode=off  EnableBusSupport=off
  Terminator : Terminator
  wires:
  EC_EEPROM_Init/1 -> EEPROM_Mirror_s/1
  EEPROM_Mirror_s/1 -> Terminator/1

== system LibEEPROM_eeprom_example_ORIGINAL/EEPROM_ReadRetain/EEPROM_retain_var_4/IO_EEPROM_GetStatus ==
  IO_EEPROM_GetStatus_s : S-Function  FunctionName=IO_EEPROM_GetStatus_s  Parameters=SampleTime  SFunctionDeploymentMode=off  EnableBusSupport=off
  ErrorCode : Outport  VectorParamsAs1DForOutWhenUnconnected=off
  wires:
  IO_EEPROM_GetStatus_s/1 -> ErrorCode/1

== system LibEEPROM_eeprom_example_ORIGINAL/EEPROM_ReadRetain/EEPROM_retain_var_4/IO_EEPROM_Init ==
  IO_EEPROM_Init_s : S-Function  FunctionName=IO_EEPROM_Init_s  Parameters=SampleTime  SFunctionDeploymentMode=off  EnableBusSupport=off
  ErrorCode : Outport  VectorParamsAs1DForOutWhenUnconnected=off
  wires:
  IO_EEPROM_Init_s/1 -> ErrorCode/1

== system LibEEPROM_eeprom_example_ORIGINAL/EEPROM_ReadRetain/EEPROM_retain_var_4/Read_Mirror ==
  Read_Mirror_s : S-Function  FunctionName=Read_Mirror_s  Parameters=SampleTime,offset,length  SFunctionDeploymentMode=off  EnableBusSupport=off
  ErrorCode_EEPROM_mirror : Outport  VectorParamsAs1DForOutWhenUnconnected=off
  data : Outport  Port=2  VectorParamsAs1DForOutWhenUnconnected=off
  wires:
  Read_Mirror_s/2 -> data/1
  Read_Mirror_s/1 -> ErrorCode_EEPROM_mirror/1

== system LibEEPROM_eeprom_example_ORIGINAL/EEPROM_ReadRetain/EEPROM_retain_var_4/once_true: Mirror filled ==
  S : Inport
  Logic : CombinatorialLogic  TruthTable=[0 ;1 ;0 ;0 ;1 ;1 ;0 ;0 ]
  Memory : Memory  InitialCondition=initial_condition  InheritSampleTime=on
  Mux : Mux  Inputs=3
  R : Constant  Value=0  OutDataTypeStr=boolean
  Q : Outport  InitialOutput=0  VectorParamsAs1DForOutWhenUnconnected=off
  wires:
  R/1 -> Mux/2
  S/1 -> Mux/1
  Logic/1 -> Memory/1, Q/1
  Mux/1 -> Logic/1
  Memory/1 -> Mux/3

== system LibEEPROM_eeprom_example_ORIGINAL/EEPROM_ReadRetain/EEPROM_retain_var_5/EEPROM_Mirror ==
  EC_EEPROM_Init : Inport
  EEPROM_Mirror_s : S-Function  FunctionName=EEPROM_Mirror_s  Parameters=SampleTime,offset,length  SFunctionDeploymentMode=off  EnableBusSupport=off
  Terminator : Terminator
  wires:
  EC_EEPROM_Init/1 -> EEPROM_Mirror_s/1
  EEPROM_Mirror_s/1 -> Terminator/1

== system LibEEPROM_eeprom_example_ORIGINAL/EEPROM_ReadRetain/EEPROM_retain_var_5/IO_EEPROM_GetStatus ==
  IO_EEPROM_GetStatus_s : S-Function  FunctionName=IO_EEPROM_GetStatus_s  Parameters=SampleTime  SFunctionDeploymentMode=off  EnableBusSupport=off
  ErrorCode : Outport  VectorParamsAs1DForOutWhenUnconnected=off
  wires:
  IO_EEPROM_GetStatus_s/1 -> ErrorCode/1

== system LibEEPROM_eeprom_example_ORIGINAL/EEPROM_ReadRetain/EEPROM_retain_var_5/IO_EEPROM_Init ==
  IO_EEPROM_Init_s : S-Function  FunctionName=IO_EEPROM_Init_s  Parameters=SampleTime  SFunctionDeploymentMode=off  EnableBusSupport=off
  ErrorCode : Outport  VectorParamsAs1DForOutWhenUnconnected=off
  wires:
  IO_EEPROM_Init_s/1 -> ErrorCode/1

== system LibEEPROM_eeprom_example_ORIGINAL/EEPROM_ReadRetain/EEPROM_retain_var_5/Read_Mirror ==
  Read_Mirror_s : S-Function  FunctionName=Read_Mirror_s  Parameters=SampleTime,offset,length  SFunctionDeploymentMode=off  EnableBusSupport=off
  ErrorCode_EEPROM_mirror : Outport  VectorParamsAs1DForOutWhenUnconnected=off
  data : Outport  Port=2  VectorParamsAs1DForOutWhenUnconnected=off
  wires:
  Read_Mirror_s/2 -> data/1
  Read_Mirror_s/1 -> ErrorCode_EEPROM_mirror/1

== system LibEEPROM_eeprom_example_ORIGINAL/EEPROM_ReadRetain/EEPROM_retain_var_5/once_true: Mirror filled ==
  S : Inport
  Logic : CombinatorialLogic  TruthTable=[0 ;1 ;0 ;0 ;1 ;1 ;0 ;0 ]
  Memory : Memory  InitialCondition=initial_condition  InheritSampleTime=on
  Mux : Mux  Inputs=3
  R : Constant  Value=0  OutDataTypeStr=boolean
  Q : Outport  InitialOutput=0  VectorParamsAs1DForOutWhenUnconnected=off
  wires:
  R/1 -> Mux/2
  S/1 -> Mux/1
  Logic/1 -> Memory/1, Q/1
  Mux/1 -> Logic/1
  Memory/1 -> Mux/3

== system LibEEPROM_eeprom_example_ORIGINAL/EEPROM_WriteParam1/EEPROM_CRC_OK/EEPROM_Mirror ==
  EC_EEPROM_Init : Inport
  EEPROM_Mirror_s : S-Function  FunctionName=EEPROM_Mirror_s  Parameters=SampleTime,offset,length  SFunctionDeploymentMode=off  EnableBusSupport=off
  Terminator : Terminator
  wires:
  EC_EEPROM_Init/1 -> EEPROM_Mirror_s/1
  EEPROM_Mirror_s/1 -> Terminator/1

== system LibEEPROM_eeprom_example_ORIGINAL/EEPROM_WriteParam1/EEPROM_CRC_OK/IO_EEPROM_GetStatus ==
  IO_EEPROM_GetStatus_s : S-Function  FunctionName=IO_EEPROM_GetStatus_s  Parameters=SampleTime  SFunctionDeploymentMode=off  EnableBusSupport=off
  ErrorCode : Outport  VectorParamsAs1DForOutWhenUnconnected=off
  wires:
  IO_EEPROM_GetStatus_s/1 -> ErrorCode/1

== system LibEEPROM_eeprom_example_ORIGINAL/EEPROM_WriteParam1/EEPROM_CRC_OK/IO_EEPROM_GetStatus2 ==
  IO_EEPROM_GetStatus_s : S-Function  FunctionName=IO_EEPROM_GetStatus_s  Parameters=SampleTime  SFunctionDeploymentMode=off  EnableBusSupport=off
  ErrorCode : Outport  VectorParamsAs1DForOutWhenUnconnected=off
  wires:
  IO_EEPROM_GetStatus_s/1 -> ErrorCode/1

== system LibEEPROM_eeprom_example_ORIGINAL/EEPROM_WriteParam1/EEPROM_CRC_OK/IO_EEPROM_Init ==
  IO_EEPROM_Init_s : S-Function  FunctionName=IO_EEPROM_Init_s  Parameters=SampleTime  SFunctionDeploymentMode=off  EnableBusSupport=off
  ErrorCode : Outport  VectorParamsAs1DForOutWhenUnconnected=off
  wires:
  IO_EEPROM_Init_s/1 -> ErrorCode/1

== system LibEEPROM_eeprom_example_ORIGINAL/EEPROM_WriteParam1/EEPROM_CRC_OK/IO_EEPROM_Write_ALL ==
  EC_Write_Mirror : Inport
  GetStatus : Inport  Port=2
  IO_EEPROM_Write_s : S-Function  FunctionName=IO_EEPROM_Write_s  Parameters=SampleTime,offset,length  SFunctionDeploymentMode=off  EnableBusSupport=off
  ErrorCode : Outport  VectorParamsAs1DForOutWhenUnconnected=off
  wires:
  EC_Write_Mirror/1 -> IO_EEPROM_Write_s/1
  GetStatus/1 -> IO_EEPROM_Write_s/2
  IO_EEPROM_Write_s/1 -> ErrorCode/1

== system LibEEPROM_eeprom_example_ORIGINAL/EEPROM_WriteParam1/EEPROM_CRC_OK/Write_Mirror ==
  b_trigger : Inport
  data : Inport  Port=2
  Write_Mirror_s : S-Function  FunctionName=Write_Mirror_s  Parameters=SampleTime,offset,length  SFunctionDeploymentMode=off  EnableBusSupport=off
  ErrorCode_EEPROM_mirror : Outport  VectorParamsAs1DForOutWhenUnconnected=off
  wires:
  b_trigger/1 -> Write_Mirror_s/1
  data/1 -> Write_Mirror_s/2
  Write_Mirror_s/1 -> ErrorCode_EEPROM_mirror/1

== system LibEEPROM_eeprom_example_ORIGINAL/EEPROM_WriteParam1/EEPROM_CRC_OK/crc32_calc_intern ==
  Trigger : TriggerPort  VariantControl=(inherit)
  crc32_calc_intern_s : S-Function  FunctionName=crc32_calc_intern_s  Parameters=SampleTime,EEPROM_mirror,iBasicAddr_intern,iEndAddr_intern  SFunctionDeploymentMode=off  EnableBusSupport=off
  ErrorCode : Outport  VectorParamsAs1DForOutWhenUnconnected=off
  crc32 : Outport  Port=2  VectorParamsAs1DForOutWhenUnconnected=off
  wires:
  crc32_calc_intern_s/2 -> crc32/1
  crc32_calc_intern_s/1 -> ErrorCode/1

== system LibEEPROM_eeprom_example_ORIGINAL/EEPROM_WriteParam1/EEPROM_param_1/Write_Mirror ==
  b_trigger : Inport
  data : Inport  Port=2
  Write_Mirror_s : S-Function  FunctionName=Write_Mirror_s  Parameters=SampleTime,offset,length  SFunctionDeploymentMode=off  EnableBusSupport=off
  ErrorCode_EEPROM_mirror : Outport  VectorParamsAs1DForOutWhenUnconnected=off
  wires:
  Write_Mirror_s/1 -> ErrorCode_EEPROM_mirror/1
  data/1 -> Write_Mirror_s/2
  b_trigger/1 -> Write_Mirror_s/1

== system LibEEPROM_eeprom_example_ORIGINAL/EEPROM_WriteParam1/EEPROM_param_2/Write_Mirror ==
  b_trigger : Inport
  data : Inport  Port=2
  Write_Mirror_s : S-Function  FunctionName=Write_Mirror_s  Parameters=SampleTime,offset,length  SFunctionDeploymentMode=off  EnableBusSupport=off
  ErrorCode_EEPROM_mirror : Outport  VectorParamsAs1DForOutWhenUnconnected=off
  wires:
  Write_Mirror_s/1 -> ErrorCode_EEPROM_mirror/1
  data/1 -> Write_Mirror_s/2
  b_trigger/1 -> Write_Mirror_s/1

== system LibEEPROM_eeprom_example_ORIGINAL/EEPROM_WriteParam1/EEPROM_param_3/Write_Mirror ==
  b_trigger : Inport
  data : Inport  Port=2
  Write_Mirror_s : S-Function  FunctionName=Write_Mirror_s  Parameters=SampleTime,offset,length  SFunctionDeploymentMode=off  EnableBusSupport=off
  ErrorCode_EEPROM_mirror : Outport  VectorParamsAs1DForOutWhenUnconnected=off
  wires:
  Write_Mirror_s/1 -> ErrorCode_EEPROM_mirror/1
  data/1 -> Write_Mirror_s/2
  b_trigger/1 -> Write_Mirror_s/1

== system LibEEPROM_eeprom_example_ORIGINAL/EEPROM_WriteParam1/EEPROM_param_4/Write_Mirror ==
  b_trigger : Inport
  data : Inport  Port=2
  Write_Mirror_s : S-Function  FunctionName=Write_Mirror_s  Parameters=SampleTime,offset,length  SFunctionDeploymentMode=off  EnableBusSupport=off
  ErrorCode_EEPROM_mirror : Outport  VectorParamsAs1DForOutWhenUnconnected=off
  wires:
  Write_Mirror_s/1 -> ErrorCode_EEPROM_mirror/1
  data/1 -> Write_Mirror_s/2
  b_trigger/1 -> Write_Mirror_s/1

== system LibEEPROM_eeprom_example_ORIGINAL/EEPROM_WriteParam1/EEPROM_param_5/Write_Mirror ==
  b_trigger : Inport
  data : Inport  Port=2
  Write_Mirror_s : S-Function  FunctionName=Write_Mirror_s  Parameters=SampleTime,offset,length  SFunctionDeploymentMode=off  EnableBusSupport=off
  ErrorCode_EEPROM_mirror : Outport  VectorParamsAs1DForOutWhenUnconnected=off
  wires:
  Write_Mirror_s/1 -> ErrorCode_EEPROM_mirror/1
  data/1 -> Write_Mirror_s/2
  b_trigger/1 -> Write_Mirror_s/1

== system LibEEPROM_eeprom_example_ORIGINAL/EEPROM_WriteParam1/EEPROM_param_6/Write_Mirror ==
  b_trigger : Inport
  data : Inport  Port=2
  Write_Mirror_s : S-Function  FunctionName=Write_Mirror_s  Parameters=SampleTime,offset,length  SFunctionDeploymentMode=off  EnableBusSupport=off
  ErrorCode_EEPROM_mirror : Outport  VectorParamsAs1DForOutWhenUnconnected=off
  wires:
  Write_Mirror_s/1 -> ErrorCode_EEPROM_mirror/1
  data/1 -> Write_Mirror_s/2
  b_trigger/1 -> Write_Mirror_s/1
